simulink model "Pitch_simulink_lqr"  (R2018b)
settings: Solver=VariableStepAuto  StartTime=0.0  StopTime=7  RelTol=1e-3
values from neighbouring files (symbols this model uses):
  Ap = [0,1;0,sin(beta)/Iyy*(N^2/int_resist+c)*(-2*sin(beta)-Iyy/(Iw*sin(beta)))]    [Spacecraft.m]
  beta = 63.4*pi/180    (= 1.10653874576)    [Spacecraft.m]
  Bp = [0;sin(beta)*N/(Iyy*int_resist)]    [Spacecraft.m]
  Cp = [1,0;0,1]    [Spacecraft.m]
  Dp = [0;0]    [Spacecraft.m]
  int_resist = 6    [Spacecraft.m]
  Iw = max([Iw_roll Iw_pitch Iw_yaw])    [Spacecraft.m]    (also in maneuver.m = z2(end)*Is/(4*Omega_max*cos(beta)))
  Iyy = 50000    [Spacecraft.m]
  Kp = lqr(Ap,Bp,Qp,Rp)    [Spacecraft.m]
  N = 60    [Spacecraft.m]
  pitch_overshoot = 0.05    [Spacecraft.m]
libraries: simulink x1
settings Model: Creator=Utilisateur  LastModifiedBy=Utilisateur

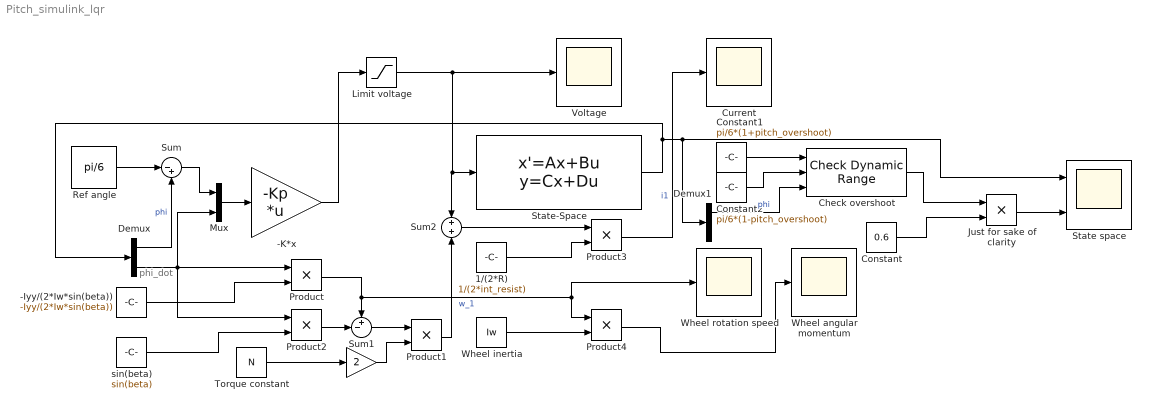
== system Pitch_simulink_lqr ==
  note: phi_dot
  " " : Gain  Gain=2
  -Iyy/(2*Iw*sin(beta)) : Constant  Value=-Iyy/(2*Iw*sin(beta))
  "-K*x " : Gain  Gain=-Kp  Multiplication=Matrix(K*u) (u vector)
  1/(2*R) : Constant  Value=1/(2*int_resist)
  Check overshoot : simulink/Model Verification/Check  Dynamic Range  Description=min < u < max  enabled=on  stopWhenAssertionFail=off  export=on  icon=graphic
      settings: SourceProductName=Simulink  SourceProductBaseCode=SL
  Constant : Constant  Value=0.6
  Constant1 : Constant  Value=pi/6*(1+pitch_overshoot)
  Constant2 : Constant  Value=pi/6*(1-pitch_overshoot)
  Current : Scope
  Demux : Demux  Outputs=2
  Demux1 : Demux  Outputs=2
  Just for sake of clarity : Product
  Limit voltage : Saturate  UpperLimit=600  LowerLimit=-600
  Mux : Mux  Inputs=2
  Product{,1..4} (5 alike) : Product
  Ref angle : Constant  Value=pi/6
  State space : Scope  NumInputPorts=2
  State-Space : StateSpace  A=Ap  B=Bp  C=Cp  D=Dp  InitialCondition=[0;0]
  Sum : Sum  Inputs=|-+
  Sum1 : Sum  Inputs=+-|
  Sum2 : Sum  Inputs=+|+
  Torque constant : Constant  Value=N
  Voltage : Scope
  Wheel angular momentum : Scope
  Wheel inertia : Constant  Value=Iw
  Wheel rotation speed : Scope
  sin(beta) : Constant  Value=sin(beta)
  wires:
  Wheel inertia/1 -> Product4/2
  Product/1 -> Product4/1, Wheel rotation speed/1, Sum1/1  "w_1"
  Ref angle/1 -> Sum/1
  Limit voltage/1 -> Sum2/1, State-Space/1, Voltage/1
  Demux/2 -> Product/1, Mux/2, Product2/1
  -Iyy/(2*Iw*sin(beta))/1 -> Product/2
  Product4/1 -> Wheel angular momentum/1
  1/(2*R)/1 -> Product3/2
  Demux/1 -> Sum/2  "phi"
  sin(beta)/1 -> Product2/2
  State-Space/1 -> Demux1/1, State space/1, Demux/1
  " "/1 -> Product1/2
  Mux/1 -> "-K*x "/1
  Torque constant/1 -> " "/1
  Sum/1 -> Mux/1
  Sum2/1 -> Product3/1
  Product2/1 -> Sum1/2
  "-K*x "/1 -> Limit voltage/1
  Product1/1 -> Sum2/2
  Sum1/1 -> Product1/1
  Product3/1 -> Current/1  "i1"
  Demux1/1 -> Check overshoot/3  "phi"
  Check overshoot/1 -> Just for sake of clarity/1
  Constant1/1 -> Check overshoot/1
  Constant/1 -> Just for sake of clarity/2
  Just for sake of clarity/1 -> State space/2
  Constant2/1 -> Check overshoot/2
